simulink model "Controller"  (R2022b)
settings: Solver=VariableStepAuto  StartTime=0.0  StopTime=15*3600  RelTol=1e-3
model workspace (MAT data in the model file):
  J = 8.6
  Kd = 5
  Kf = 0.07
  Kg = 2000
  Kt = 0.07
  L = 1e-05
  R = 10
libraries: slpidlib x2
settings Model: Creator=adlercohen  LastModifiedBy=adlercohen
settings DataIOCC: ExternalInput=[sunTime, sunElevation, sunPosition]  LoadExternalInput=on

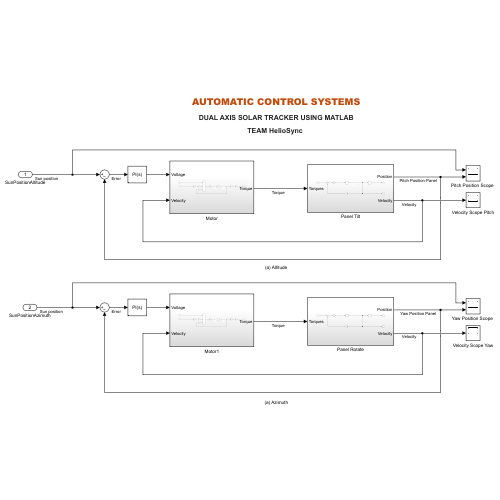
[thumbnail: Simulink's stored preview of the top-level diagram]
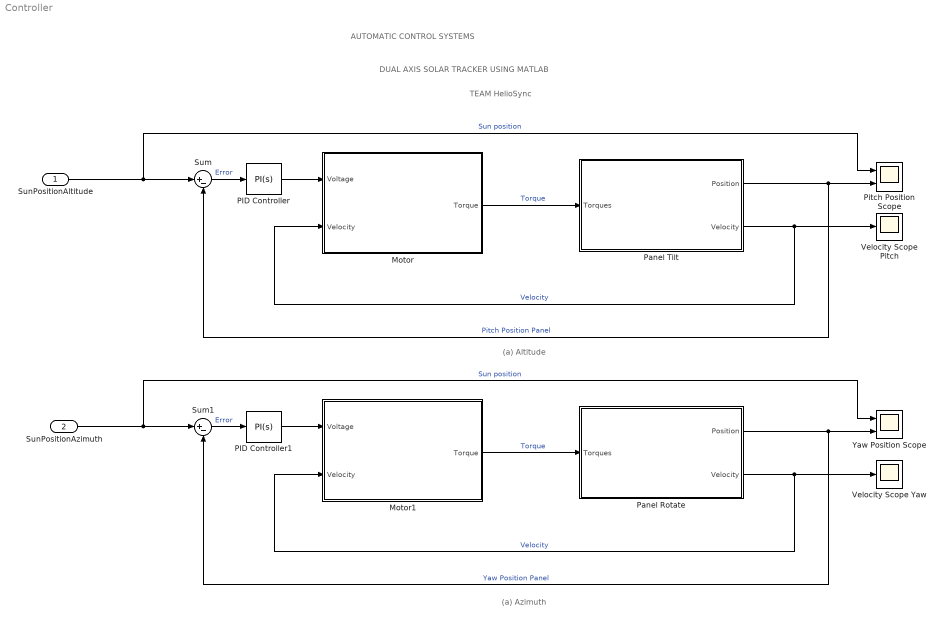
== system Controller ==
  note: DUAL AXIS SOLAR TRACKER USING MATLAB
  note: AUTOMATIC CONTROL SYSTEMS
  note: (a) Altitude
  note: (a) Azimuth
  note: TEAM HelioSync
  SunPositionAltitude : Inport
  SunPositionAzimuth : Inport  Port=2
  Motor : Subsystem
  Motor1 : Subsystem
  PID Controller : slpidlib/PID Controller  Controller=PI  Form=Parallel  TimeDomain=Continuous-time  UseExternalTs=off  SampleTime=-1  IntegratorMethod=Forward Euler  FilterMethod=Forward Euler  ControllerParametersSource=internal  P=240  I=180  UseKiTs=off  D=0  N=100  UseFilter=on  TunerSelectOption=Transfer Function Based (PID Tuner App)  InitialConditionSource=internal  InitialConditionForIntegrator=0  InitialConditionForFilter=0  DifferentiatorICPrevScaledInput=0  ExternalReset=none  TrackingMode=off  Kt=1  LimitOutput=off  SatLimitsSource=internal  UpperSaturationLimit=inf  LowerSaturationLimit=-inf  LinearizeAsGain=on  AntiWindupMode=none  Kb=1  LimitIntegrator=off  UpperIntegratorSaturationLimit=inf  LowerIntegratorSaturationLimit=-inf  POutMin=[]  POutMax=[]  IOutMin=[]  IOutMax=[]  DOutMin=[]  DOutMax=[]  NOutMin=[]  NOutMax=[]  SumOutMin=[]  SumOutMax=[]  SaturationOutMin=[]  SaturationOutMax=[]  PParamMin=[]  PParamMax=[]  IParamMin=[]  IParamMax=[]  DParamMin=[]  DParamMax=[]  NParamMin=[]  NParamMax=[]  KbParamMin=[]  KbParamMax=[]  KtParamMin=[]  KtParamMax=[]  KbOutMin=[]  KbOutMax=[]  KtOutMin=[]  KtOutMax=[]  IntegratorOutMin=[]  IntegratorOutMax=[]  FilterOutMin=[]  FilterOutMax=[]  SumI1OutMin=[]  SumI1OutMax=[]  SumI2OutMin=[]  SumI2OutMax=[]  SumI3OutMin=[]  SumI3OutMax=[]  SumI4OutMin=[]  SumI4OutMax=[]  SumDOutMin=[]  SumDOutMax=[]  DifferentiatorOutMin=[]  DifferentiatorOutMax=[]  FilterDiffOutCoefMin=[]  FilterDiffOutCoefMax=[]  ReciprocalOutMin=[]  ReciprocalOutMax=[]  SumDenOutMin=[]  SumDenOutMax=[]  SumNumOutMin=[]  SumNumOutMax=[]  DivideOutMin=[]  DivideOutMax=[]  UdiffTsProdOutMin=[]  UdiffTsProdOutMax=[]  NTsProdOutMin=[]  NTsProdOutMax=[]  UintegralTsProdOutMin=[]  UintegralTsProdOutMax=[]  UngainTsProdOutMin=[]  UngainTsProdOutMax=[]  ClampingZeroOutDataTypeStr=Inherit: Inherit via back propagation  ClampingZeroOutMin=[]  ClampingZeroOutMax=[]  FilterDenConstantOutDataTypeStr=Inherit: Inherit via back propagation  FilterDenConstantOutMin=[]  FilterDenConstantOutMax=[]  PCopyOutDataTypeStr=Inherit: Inherit via back propagation  PCopyOutMin=[]  PCopyOutMax=[]  NCopyOutDataTypeStr=Inherit: Inherit via back propagation  NCopyOutMin=[]  NCopyOutMax=[]  IntegratorContinuousStateAttributes=''  IntegratorStateMustResolveToSignalObject=off  IntegratorRTWStateStorageClass=Auto  FilterContinuousStateAttributes=''  FilterStateMustResolveToSignalObject=off  FilterRTWStateStorageClass=Auto  ParallelPVariant=InternalParameters  IdealPVariant=Disabled  IVariant=InternalParameters  DVariant=Disabled  IntegratorVariant=Continuous  SatVariant=Disabled  AWVariant=Passthrough  PCopyVariant=Disabled  TRVariant=Disabled  FdbkBlocksVariant=Forward  IdealPFdbkVariant=Disabled  SatFdbkVariant=Disabled  DerivativeFilterVariant=Disabled  NVariant=Disabled  NCopyVariant=Disabled_SignalSpec  FilterICVariant=Disabled  IntegratorICVariant=InternalICs  ExternalResetVariant=Disabled  TRSumVariant=Passthrough  SumFdbkVariant=Disabled  SumVariant=Sum_PI  TsampFilterVariant=InternalTs  TsampNgainVariant=Passthrough  TsampIntegralVariant=Passthrough  ExternalSaturationOutDataTypeStr=Inherit: Same as second input
  PID Controller1 : slpidlib/PID Controller  Controller=PI  Form=Parallel  TimeDomain=Continuous-time  UseExternalTs=off  SampleTime=-1  IntegratorMethod=Forward Euler  FilterMethod=Forward Euler  ControllerParametersSource=internal  P=240  I=180  UseKiTs=off  D=0  N=100  UseFilter=on  TunerSelectOption=Transfer Function Based (PID Tuner App)  InitialConditionSource=internal  InitialConditionForIntegrator=0  InitialConditionForFilter=0  DifferentiatorICPrevScaledInput=0  ExternalReset=none  TrackingMode=off  Kt=1  LimitOutput=off  SatLimitsSource=internal  UpperSaturationLimit=inf  LowerSaturationLimit=-inf  LinearizeAsGain=on  AntiWindupMode=none  Kb=1  LimitIntegrator=off  UpperIntegratorSaturationLimit=inf  LowerIntegratorSaturationLimit=-inf  POutMin=[]  POutMax=[]  IOutMin=[]  IOutMax=[]  DOutMin=[]  DOutMax=[]  NOutMin=[]  NOutMax=[]  SumOutMin=[]  SumOutMax=[]  SaturationOutMin=[]  SaturationOutMax=[]  PParamMin=[]  PParamMax=[]  IParamMin=[]  IParamMax=[]  DParamMin=[]  DParamMax=[]  NParamMin=[]  NParamMax=[]  KbParamMin=[]  KbParamMax=[]  KtParamMin=[]  KtParamMax=[]  KbOutMin=[]  KbOutMax=[]  KtOutMin=[]  KtOutMax=[]  IntegratorOutMin=[]  IntegratorOutMax=[]  FilterOutMin=[]  FilterOutMax=[]  SumI1OutMin=[]  SumI1OutMax=[]  SumI2OutMin=[]  SumI2OutMax=[]  SumI3OutMin=[]  SumI3OutMax=[]  SumI4OutMin=[]  SumI4OutMax=[]  SumDOutMin=[]  SumDOutMax=[]  DifferentiatorOutMin=[]  DifferentiatorOutMax=[]  FilterDiffOutCoefMin=[]  FilterDiffOutCoefMax=[]  ReciprocalOutMin=[]  ReciprocalOutMax=[]  SumDenOutMin=[]  SumDenOutMax=[]  SumNumOutMin=[]  SumNumOutMax=[]  DivideOutMin=[]  DivideOutMax=[]  UdiffTsProdOutMin=[]  UdiffTsProdOutMax=[]  NTsProdOutMin=[]  NTsProdOutMax=[]  UintegralTsProdOutMin=[]  UintegralTsProdOutMax=[]  UngainTsProdOutMin=[]  UngainTsProdOutMax=[]  ClampingZeroOutDataTypeStr=Inherit: Inherit via back propagation  ClampingZeroOutMin=[]  ClampingZeroOutMax=[]  FilterDenConstantOutDataTypeStr=Inherit: Inherit via back propagation  FilterDenConstantOutMin=[]  FilterDenConstantOutMax=[]  PCopyOutDataTypeStr=Inherit: Inherit via back propagation  PCopyOutMin=[]  PCopyOutMax=[]  NCopyOutDataTypeStr=Inherit: Inherit via back propagation  NCopyOutMin=[]  NCopyOutMax=[]  IntegratorContinuousStateAttributes=''  IntegratorStateMustResolveToSignalObject=off  IntegratorRTWStateStorageClass=Auto  FilterContinuousStateAttributes=''  FilterStateMustResolveToSignalObject=off  FilterRTWStateStorageClass=Auto  ParallelPVariant=InternalParameters  IdealPVariant=Disabled  IVariant=InternalParameters  DVariant=Disabled  IntegratorVariant=Continuous  SatVariant=Disabled  AWVariant=Passthrough  PCopyVariant=Disabled  TRVariant=Disabled  FdbkBlocksVariant=Forward  IdealPFdbkVariant=Disabled  SatFdbkVariant=Disabled  DerivativeFilterVariant=Disabled  NVariant=Disabled  NCopyVariant=Disabled_SignalSpec  FilterICVariant=Disabled  IntegratorICVariant=InternalICs  ExternalResetVariant=Disabled  TRSumVariant=Passthrough  SumFdbkVariant=Disabled  SumVariant=Sum_PI  TsampFilterVariant=InternalTs  TsampNgainVariant=Passthrough  TsampIntegralVariant=Passthrough  ExternalSaturationOutDataTypeStr=Inherit: Same as second input
  Panel Rotate : Subsystem
  Panel Tilt : Subsystem
  "Pitch Position Scope " : Scope  NumInputPorts=2
  Sum : Sum  Inputs=|+-
  Sum1 : Sum  Inputs=|+-
  Velocity Scope Pitch : Scope
  Velocity Scope Yaw : Scope
  "Yaw Position Scope " : Scope  NumInputPorts=2
  wires:
  Panel Tilt/2(Velocity) -> Motor/2(Velocity), Velocity Scope Pitch/1  "Velocity"
  Panel Tilt/1(Position) -> "Pitch Position Scope "/2, Sum/2  "Pitch Position Panel"
  Motor/1(Torque) -> Panel Tilt/1(Torques)  "Torque"
  Sum/1 -> PID Controller/1  "Error"
  PID Controller/1 -> Motor/1(Voltage)
  SunPositionAltitude/1 -> "Pitch Position Scope "/1, Sum/1  "Sun position"
  SunPositionAzimuth/1 -> "Yaw Position Scope "/1, Sum1/1  "Sun position"
  PID Controller1/1 -> Motor1/1(Voltage)
  Panel Rotate/2(Velocity) -> Motor1/2(Velocity), Velocity Scope Yaw/1  "Velocity"
  Sum1/1 -> PID Controller1/1  "Error"
  Motor1/1(Torque) -> Panel Rotate/1(Torques)  "Torque"
  Panel Rotate/1(Position) -> "Yaw Position Scope "/2, Sum1/2  "Yaw Position Panel"

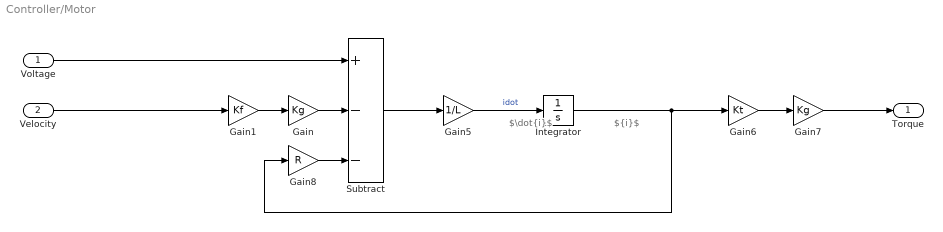
== system Controller/Motor ==
  note: $\dot{i}$
  note: ${i}$
  Voltage : Inport
  Velocity : Inport  Port=2
  Gain : Gain  Gain=Kg
  Gain1 : Gain  Gain=Kf
  Gain5 : Gain  Gain=1/L
  Gain6 : Gain  Gain=Kt
  Gain7 : Gain  Gain=Kg
  Gain8 : Gain  Gain=R
  Integrator : Integrator
  Subtract : Sum  Inputs=+--
  Torque : Outport
  wires:
  Gain/1 -> Subtract/2
  Subtract/1 -> Gain5/1
  Gain8/1 -> Subtract/3
  Integrator/1 -> Gain8/1, Gain6/1
  Gain6/1 -> Gain7/1
  Gain5/1 -> Integrator/1  "idot"
  Gain1/1 -> Gain/1
  Gain7/1 -> Torque/1
  Voltage/1 -> Subtract/1
  Velocity/1 -> Gain1/1

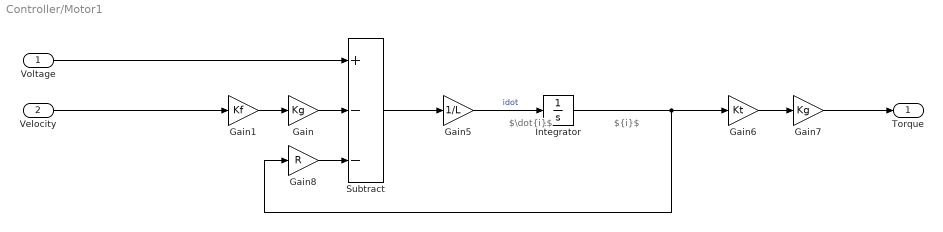
== system Controller/Motor1 ==
  note: $\dot{i}$
  note: ${i}$
  Voltage : Inport
  Velocity : Inport  Port=2
  Gain : Gain  Gain=Kg
  Gain1 : Gain  Gain=Kf
  Gain5 : Gain  Gain=1/L
  Gain6 : Gain  Gain=Kt
  Gain7 : Gain  Gain=Kg
  Gain8 : Gain  Gain=R
  Integrator : Integrator
  Subtract : Sum  Inputs=+--
  Torque : Outport
  wires:
  Gain/1 -> Subtract/2
  Subtract/1 -> Gain5/1
  Gain8/1 -> Subtract/3
  Integrator/1 -> Gain8/1, Gain6/1
  Gain6/1 -> Gain7/1
  Gain5/1 -> Integrator/1  "idot"
  Gain1/1 -> Gain/1
  Gain7/1 -> Torque/1
  Voltage/1 -> Subtract/1
  Velocity/1 -> Gain1/1

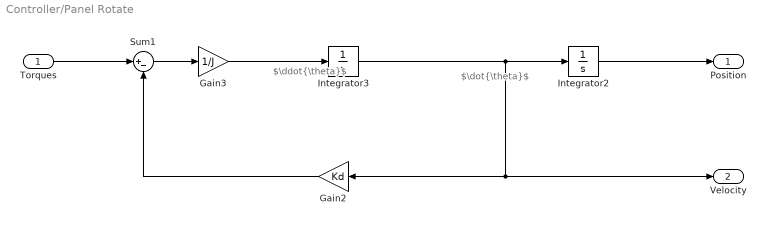
== system Controller/Panel Rotate ==
  note: $\ddot{\theta}$
  note: $\dot{\theta}$
  Torques : Inport
  Gain2 : Gain  Gain=Kd
  Gain3 : Gain  Gain=1/J
  Integrator2 : Integrator
  Integrator3 : Integrator
  Sum1 : Sum  Inputs=|+-
  Position : Outport
  Velocity : Outport  Port=2
  wires:
  Torques/1 -> Sum1/1
  Integrator3/1 -> Velocity/1, Gain2/1, Integrator2/1
  Gain2/1 -> Sum1/2
  Sum1/1 -> Gain3/1
  Integrator2/1 -> Position/1
  Gain3/1 -> Integrator3/1

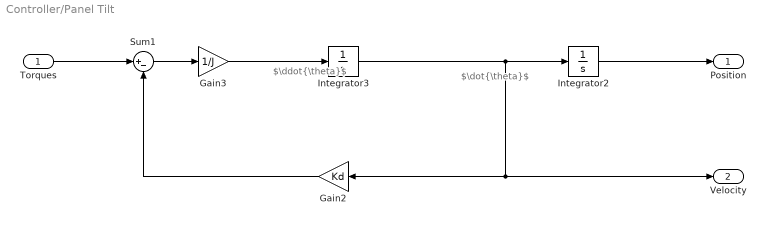
== system Controller/Panel Tilt ==
  note: $\ddot{\theta}$
  note: $\dot{\theta}$
  Torques : Inport
  Gain2 : Gain  Gain=Kd
  Gain3 : Gain  Gain=1/J
  Integrator2 : Integrator
  Integrator3 : Integrator
  Sum1 : Sum  Inputs=|+-
  Position : Outport
  Velocity : Outport  Port=2
  wires:
  Torques/1 -> Sum1/1
  Integrator3/1 -> Velocity/1, Gain2/1, Integrator2/1
  Gain2/1 -> Sum1/2
  Sum1/1 -> Gain3/1
  Integrator2/1 -> Position/1
  Gain3/1 -> Integrator3/1
